simulink model "FxLMS"  (R2018a)
settings: Solver=FixedStepDiscrete  StartTime=0.0  StopTime=5  RelTol=1e-3  EnableMultiTasking=on
undefined symbols (not defined in the file or in its folder): p_parameters, s_parameters
libraries: dspvision x3, dspindex x1
settings Model: Creator=gianc  LastModifiedBy=gianc
settings DataIOCC: LimitDataPoints=on  SaveOutput=off  SignalLogging=off  SaveTime=off
settings OptimizationCC: LifeSpan=inf
settings DebuggingCC: AlgebraicLoopMsg=error  SingleTaskRateTransMsg=error  AllowSymbolicDim=off  SFUnexpectedBacktrackingDiag=warning  SFNoUnconditionalDefaultTransitionDiag=warning  SFExecutionAtInitializationDiag=none
settings CodeAppCC: StateflowObjectComments=on
settings GRTTargetCC: TargetLangStandard=C89/C90 (ANSI)  GeneratePreprocessorConditionals=Disable all
settings ConfigComp: CovMetricSettings=dw  CovHtmlReporting=on  CovSaveCumulativeToWorkspaceVar=on  CovSaveSingleToWorkspaceVar=on  CovExternalEMLEnable=off  CovSFcnEnable=off

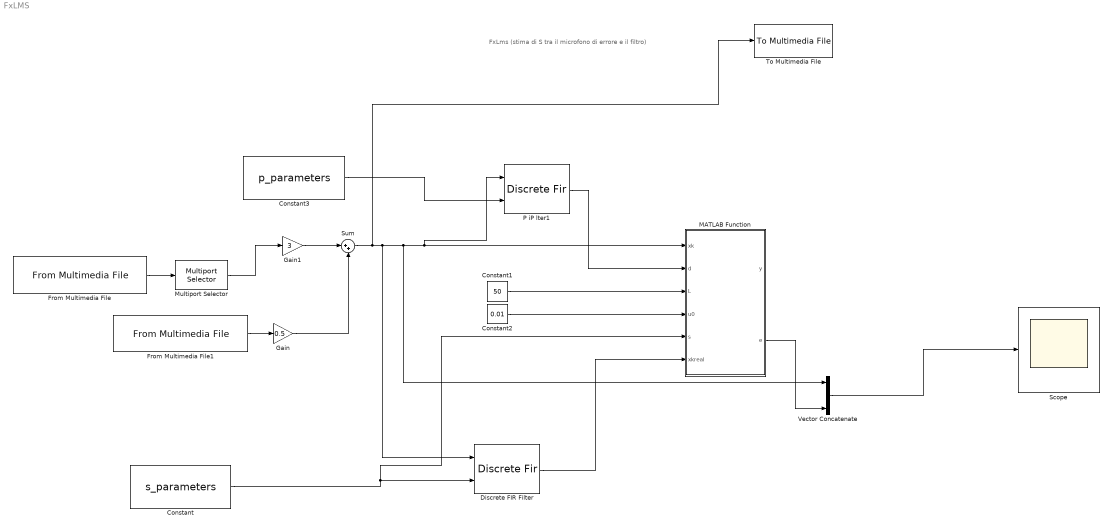
== system FxLMS ==
  note: FxLms (stima di S tra il microfono di errore e il filtro)
  Constant : Constant  Value=s_parameters  VectorParams1D=off
  Constant1 : Constant  Value=50  VectorParams1D=off
  Constant2 : Constant  Value=0.01  VectorParams1D=off
  Constant3 : Constant  Value=p_parameters  VectorParams1D=off
  Discrete FIR Filter : DiscreteFir  CoefSource=Input port  InputProcessing=Columns as channels (frame based)
      settings: InputPortMap=u0,u1
  From Multimedia File : dspvision/From Multimedia File  inputFilename=C:\Users\gianc\Downloads\gun-gunshot-01.mp3  loop=on  numPlays=10  outputStreams=Audio only  videoDataType=single  audioDataType=double  inheritSampleTime=off  userDefinedSampleTime=1/22050  noAudioOutput=off  isIntensityVideo=off  fourcc=RGB  colorVideoFormat=Separate color signals  outputEOF=off  dataOrg=Column-major  audioFrameSize=1  computeAudioFrameSize=off  outSamplingMode=Sample based
      settings: SourceProductBaseCode=VP
  From Multimedia File1 : dspvision/From Multimedia File  inputFilename=speech_dft.mp3  loop=on  numPlays=10  outputStreams=Audio only  videoDataType=single  audioDataType=double  inheritSampleTime=on  userDefinedSampleTime=1/30  noAudioOutput=off  isIntensityVideo=off  fourcc=RGB  colorVideoFormat=Separate color signals  outputEOF=off  dataOrg=Column-major  audioFrameSize=1  computeAudioFrameSize=off  outSamplingMode=Sample based
      settings: SourceProductBaseCode=VP
  Gain : Gain  Gain=0.5
  Gain1 : Gain  Gain=3
  MATLAB Function : MATLAB Function  TreatAsAtomicUnit=on
  Multiport Selector : dspindex/Multiport Selector  rowsOrCols=Columns  idxCellArray=1  idxErrMode=Clip Index
  P iP lter1 : DiscreteFir  CoefSource=Input port  InputProcessing=Columns as channels (frame based)
      settings: InputPortMap=u0,u1
  Scope : Scope
  Sum : Sum  Inputs=|++
  To Multimedia File : dspvision/To Multimedia File  outputFilename=C:\Users\gianc\Desktop\output.wav  streamSelection=Audio only  videoCompressor=None (uncompressed)  audioCompressor=None (uncompressed)  imagePorts=Separate color signals  fileType=WAV  audioDatatype=16-bit integer  fourcc=RGB  videoQuality=75  mj2000CompFactor=10
      settings: SourceProductName=Computer Vision System Toolbox  SourceProductBaseCode=VP
  Vector Concatenate : Concatenate  NumInputs=3
  wires:
  Constant1/1 -> MATLAB Function/3(L)
  Constant2/1 -> MATLAB Function/4(u0)
  From Multimedia File1/1 -> Gain/1
  Gain/1 -> Sum/2
  Gain1/1 -> Sum/1
  Vector Concatenate/1 -> Scope/1
  Constant/1 -> MATLAB Function/5(s), Discrete FIR Filter/2
  From Multimedia File/1 -> Multiport Selector/1
  Multiport Selector/1 -> Gain1/1
  Discrete FIR Filter/1 -> MATLAB Function/6(xkreal)
  P iP lter1/1 -> MATLAB Function/2(d)
  Sum/1 -> To Multimedia File/1, Discrete FIR Filter/1, Vector Concatenate/1, P iP lter1/1, MATLAB Function/1(xk)
  MATLAB Function/2(e) -> Vector Concatenate/3
  Constant3/1 -> P iP lter1/2

== matlab function FxLMS/MATLAB Function ==
  data: y output; xk input; d input; L input; u0 input; e output; s input; xkreal input
%y=output filter (anti noise)
%w=weights vector 1xL
%x=input vector 1xL
%xk=sampled input at time k
%d=wanted signal (ideal is x but we have d=P*x)

function [y,e] = fxLMS(xk,d,L,u0,s,xkreal)

%global variables
[sizeD,~]=size(d);
y=zeros(sizeD,1);
yreal=zeros(sizeD,1);
%yneg=zeros(sizeD,1);
u=u0;
e=zeros(sizeD,1);
alpha=0.1;
persistent cnt
persistent x
persistent xreal
persistent w

for i=1:sizeD
    
if isempty(cnt)
    cnt=1;
else
    cnt=cnt+1;
end

if isempty(x)
    x=zeros(1,L);
end

if isempty(xreal)
    xreal=zeros(1,L);
end

if isempty(w)
    w=zeros(1,L);
end

%calculate u opt
if cnt<=L
    u=u0;
else
    if cnt==L
        u = max(u0,alpha/(xreal*(xreal')));
    else
        u = alpha/max(u/alpha,xreal*(xreal'));
    end
end  
u;
%LMS
xreal=[xkreal(i,1) xreal(1:(L-1))];%shift and add xkreal
x=[xk(i,1) x(1:(L-1))]; %shift and add xk (FIFO)
y(i)= w*(x'); %filter adapted

% yreal = convolution(y(i),s)
[~,sizeS]=size(s);
y_volatile=y(i)*ones(1,sizeS);
yreal(i)=y_volatile*(s');
e(i) = d(i,1)-yreal(i); % e measured with a sensor or estimated
w = w + u*xreal*e(i); %refresh w for the next iteration (LMS core)
%yneg(i)=0-y(i);
end
end
